simulink model "updown_sfun_bad"  (Simulink 8.7)
settings: Solver=FixedStepDiscrete  StartTime=0.0  StopTime=10.0  RelTol=1e-3
undefined symbols (not defined in the file or in its folder): sldvsubsys
libraries: sldvlib x12, simulink x2
settings DataIOCC: LimitDataPoints=off  SaveFormat=Dataset
settings DebuggingCC: UnderspecifiedInitializationDetection=Simplified  MergeDetectMultiDrivingBlocksExec=error
settings HardwareCC: ProdBitPerPointer=64  ProdLargestAtomicFloat=Float  ProdIntDivRoundTo=Zero  ProdEndianess=LittleEndian  ProdWordSize=64  ProdHWDeviceType=Intel->x86-64 (Windows64)
settings ModelReferenceCC: PropagateSignalLabelsOutOfModel=on
settings ConfigComp: CovModelRefEnable=off

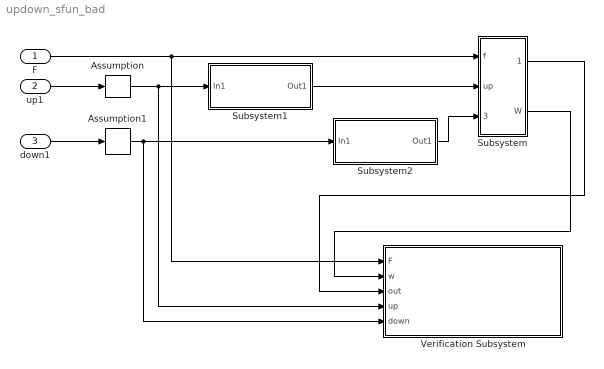
== system updown_sfun_bad ==
  F : Inport  OutDataTypeStr=boolean
  up1 : Inport  Port=2  OutDataTypeStr=int32
  down1 : Inport  Port=3  OutDataTypeStr=int32
  Assumption : sldvlib/Objectives and Constraints/Assumption  enabled=on  customAVTBlockType=Assumption  intervals=[1 60]  initial=off  dispValues=on  outEnabled=on
      settings: AttributesFormatString=%<intervals>
  Assumption1 : sldvlib/Objectives and Constraints/Assumption  enabled=on  customAVTBlockType=Assumption  intervals=[1 20]  initial=off  dispValues=on  outEnabled=on
      settings: AttributesFormatString=%<intervals>
  Subsystem : Subsystem
  Subsystem1 : Subsystem
  Subsystem2 : Subsystem
  Verification Subsystem : Subsystem  Tag=VerificationSubsystem  DisableCoverage=on  LoadFcn=sldvsubsys('check')  TreatAsAtomicUnit=on  SimViewingDevice=on  mask(VerificationSubsystem){}
      mask init:
      | sldvsubsys('maskInit');
      settings: CopyFcn=sldvsubsys('copy');  OpenFcn=open_system(gcb,'force');
      settings: PreSaveFcn=|
      | set_param(gcb,'SimViewingDevice','on');
      | sldvsubsys('check');
      mask Help: helpview(fullfile(docroot,'toolbox','sldv','sldv.map'),'verificationsubsystem')
      mask Display: image(imread('sldvicon_versubsys.png','BackGroundColor',[1 1 1]),'center');
  wires:
  Subsystem/2(W) -> Verification Subsystem/2(w)
  up1/1 -> Assumption/1
  down1/1 -> Assumption1/1
  Assumption/1 -> Verification Subsystem/4(up), Subsystem1/1(In1)
  Assumption1/1 -> Subsystem2/1(In1), Verification Subsystem/5(down)
  Subsystem2/1(Out1) -> Subsystem/3(down)
  Subsystem1/1(Out1) -> Subsystem/2(up)
  F/1 -> Verification Subsystem/1(F), Subsystem/1(f)
  Subsystem/1(Out1) -> Verification Subsystem/3(out)

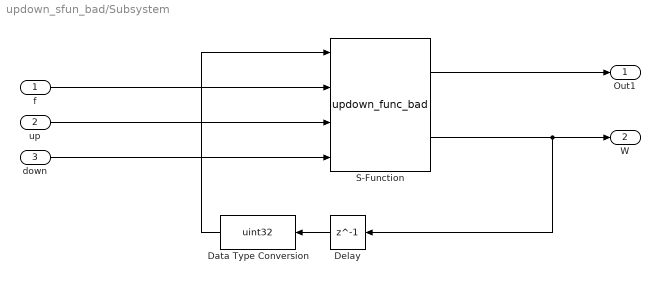
== system updown_sfun_bad/Subsystem ==
  f : Inport  OutDataTypeStr=boolean
  up : Inport  Port=2
  down : Inport  Port=3
  Data Type Conversion : DataTypeConversion  OutDataTypeStr=uint32
  Delay : Delay  DelayLength=1  InitialCondition=0
  S-Function : S-Function  FunctionName=updown_func_bad  SFunctionModules=updown_func_bad  SFunctionDeploymentMode=off  EnableBusSupport=off
  Out1 : Outport
  W : Outport  Port=2
  wires:
  S-Function/2 -> Delay/1, W/1
  Delay/1 -> Data Type Conversion/1
  Data Type Conversion/1 -> S-Function/1
  f/1 -> S-Function/2
  S-Function/1 -> Out1/1
  down/1 -> S-Function/4
  up/1 -> S-Function/3

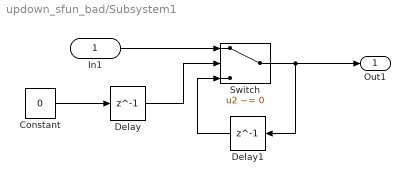
== system updown_sfun_bad/Subsystem1 ==
  In1 : Inport
  Constant : Constant  Value=0
  Delay : Delay  DelayLength=1  InitialCondition=1
  Delay1 : Delay  DelayLength=1  InitialCondition=0
  Switch : Switch  Criteria=u2 ~= 0
  Out1 : Outport
  wires:
  Delay/1 -> Switch/2
  Constant/1 -> Delay/1
  In1/1 -> Switch/1
  Switch/1 -> Delay1/1, Out1/1
  Delay1/1 -> Switch/3

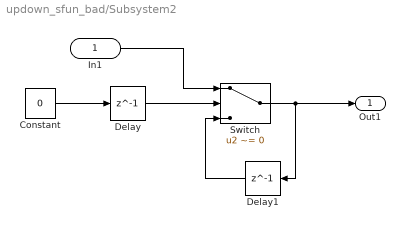
== system updown_sfun_bad/Subsystem2 ==
  In1 : Inport
  Constant : Constant  Value=0
  Delay : Delay  DelayLength=1  InitialCondition=1
  Delay1 : Delay  DelayLength=1  InitialCondition=0
  Switch : Switch  Criteria=u2 ~= 0
  Out1 : Outport
  wires:
  Delay/1 -> Switch/2
  Constant/1 -> Delay/1
  In1/1 -> Switch/1
  Switch/1 -> Out1/1, Delay1/1
  Delay1/1 -> Switch/3

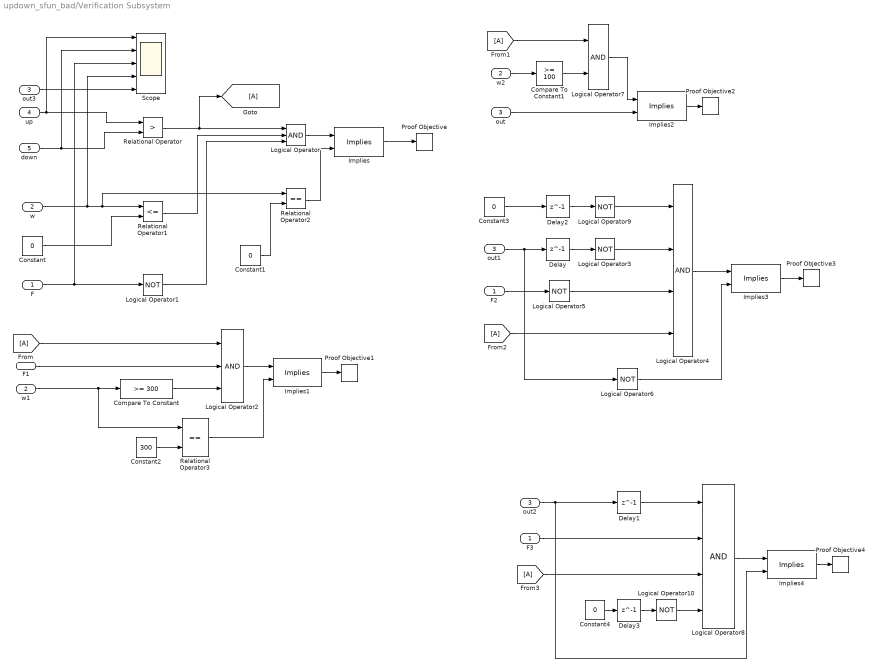
== system updown_sfun_bad/Verification Subsystem ==
  F : Inport
  w : Inport  Port=2
  out : Inport  Port=3
  up : Inport  Port=4
  down : Inport  Port=5
  Compare To Constant : simulink/Logic and Bit Operations/Compare To Constant  relop=>=  const=300  OutDataTypeStr=boolean
  Compare To Constant1 : simulink/Logic and Bit Operations/Compare To Constant  relop=>=  const=100  OutDataTypeStr=boolean
  Constant{,1,3..4} (4 alike) : Constant  Value=0
  Constant2 : Constant  Value=300
  Delay : Delay  DelayLength=1  InitialCondition=0
  Delay1 : Delay  DelayLength=1  InitialCondition=0
  Delay2 : Delay  DelayLength=1  InitialCondition=1
  Delay3 : Delay  DelayLength=1  InitialCondition=1
  F1 : InportShadow
  F2 : InportShadow
  F3 : InportShadow
  Implies{,1..4} (5 alike) : sldvlib/Verification Utilities/Implies
  Logical Operator : Logic  Inputs=3  AllPortsSameDT=off  OutDataTypeStr=boolean
  Logical Operator{1,3,5..6,9..10} (6 alike) : Logic  Operator=NOT  Inputs=3  AllPortsSameDT=off  OutDataTypeStr=boolean
  Logical Operator2 : Logic  Inputs=3  AllPortsSameDT=off  OutDataTypeStr=boolean
  Logical Operator4 : Logic  Inputs=4  AllPortsSameDT=off  OutDataTypeStr=boolean
  Logical Operator7 : Logic  AllPortsSameDT=off  OutDataTypeStr=boolean
  Logical Operator8 : Logic  Inputs=4  AllPortsSameDT=off  OutDataTypeStr=boolean
  Proof Objective{,1..2,4} (4 alike) : sldvlib/Objectives and Constraints/Proof Objective  enabled=on  customAVTBlockType=Proof Objective  intervals=true  dispValues=on  outEnabled=off  enableStopSim=on
      settings: AttributesFormatString=%<intervals>
  Proof Objective3 : sldvlib/Objectives and Constraints/Proof Objective  enabled=on  customAVTBlockType=Proof Objective  intervals=true  dispValues=on  outEnabled=off  enableStopSim=off
      settings: AttributesFormatString=%<intervals>
  Relational Operator : RelationalOperator  Operator=>  OutDataTypeStr=boolean
  Relational Operator1 : RelationalOperator  Operator=<=  OutDataTypeStr=boolean
  Relational Operator2 : RelationalOperator  Operator===  OutDataTypeStr=boolean
  Relational Operator3 : RelationalOperator  Operator===  OutDataTypeStr=boolean
  Scope : Scope  NumInputPorts=5
  out1 : InportShadow  Port=3
  out2 : InportShadow  Port=3
  out3 : InportShadow  Port=3
  w1 : InportShadow  Port=2
  w2 : InportShadow  Port=2
  wires:
  down/1 -> Relational Operator/2, Scope/2
  out3/1 -> Scope/5
  [A] -> Logical Operator7/1
  Logical Operator7/1 -> Implies2/1
  [A] -> Logical Operator8/3
  [A] -> Logical Operator4/4
  F3/1 -> Logical Operator8/2
  out2/1 -> Delay1/1, Implies4/2
  Logical Operator8/1 -> Implies4/1
  Implies4/1 -> Proof Objective4/1
  Delay1/1 -> Logical Operator8/1
  Logical Operator6/1 -> Implies3/2
  Logical Operator4/1 -> Implies3/1
  Implies3/1 -> Proof Objective3/1
  F2/1 -> Logical Operator5/1
  Delay/1 -> Logical Operator3/1
  out1/1 -> Delay/1, Logical Operator6/1
  Compare To Constant1/1 -> Logical Operator7/2
  w2/1 -> Compare To Constant1/1
  out/1 -> Implies2/2
  Implies2/1 -> Proof Objective2/1
  F1/1 -> Logical Operator2/2
  Compare To Constant/1 -> Logical Operator2/3
  w1/1 -> Compare To Constant/1, Relational Operator3/1
  Implies1/1 -> Proof Objective1/1
  Relational Operator3/1 -> Implies1/2
  Constant2/1 -> Relational Operator3/2
  Logical Operator2/1 -> Implies1/1
  [A] -> Logical Operator2/1
  Implies/1 -> Proof Objective/1
  Relational Operator2/1 -> Implies/2
  Constant1/1 -> Relational Operator2/2
  Logical Operator/1 -> Implies/1
  Logical Operator1/1 -> Logical Operator/3
  F/1 -> Logical Operator1/1, Scope/3
  Relational Operator1/1 -> Logical Operator/2
  Relational Operator/1 -> Logical Operator/1, [A]
  Constant/1 -> Relational Operator1/2
  w/1 -> Relational Operator1/1, Relational Operator2/1, Scope/4
  up/1 -> Relational Operator/1, Scope/1
  Constant3/1 -> Delay2/1
  Delay2/1 -> Logical Operator9/1
  Constant4/1 -> Delay3/1
  Delay3/1 -> Logical Operator10/1
  Logical Operator10/1 -> Logical Operator8/4
  Logical Operator9/1 -> Logical Operator4/1
  Logical Operator5/1 -> Logical Operator4/3
  Logical Operator3/1 -> Logical Operator4/2
